simulink model "Automatic_Power_Factor_Improvement_of_Induction_Motor"  (R2022b)
settings: Solver=VariableStepAuto  StartTime=0.0  StopTime=60  RelTol=1e-3
libraries: spsSeriesRLCLoadLib x10, spsIdealSwitchLib x9, spsSeriesRLCBranchLib x4, spsACVoltageSourceLib x1, spsCurrentMeasurementLib x1, spsPowerLib x1, spsVoltageMeasurementLib x1, spspowerguiLib x1
settings Model: PacingRate=0.100000  Creator=saman  LastModifiedBy=MaL!Th
settings SolverCC: ZeroCrossAlgorithm=Adaptive
settings DebuggingCC: IgnoredZcDiagnostic=none  UnconnectedInputMsg=warning  UnconnectedOutputMsg=warning  UnconnectedLineMsg=warning
settings ModelReferenceCC: EnableRefExpFcnMdlSchedulingChecks=on
settings RTWCC: DLArmComputeVersion=19.05

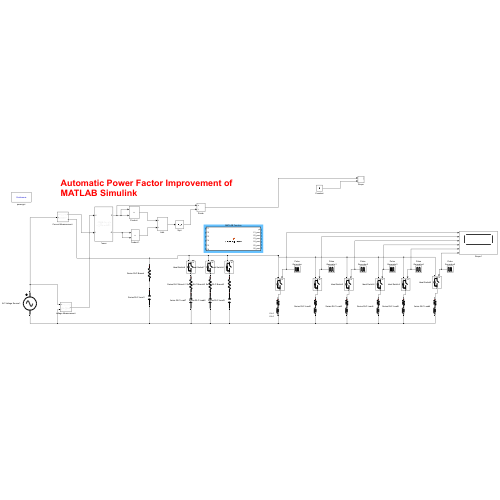
[thumbnail: Simulink's stored preview of the top-level diagram]
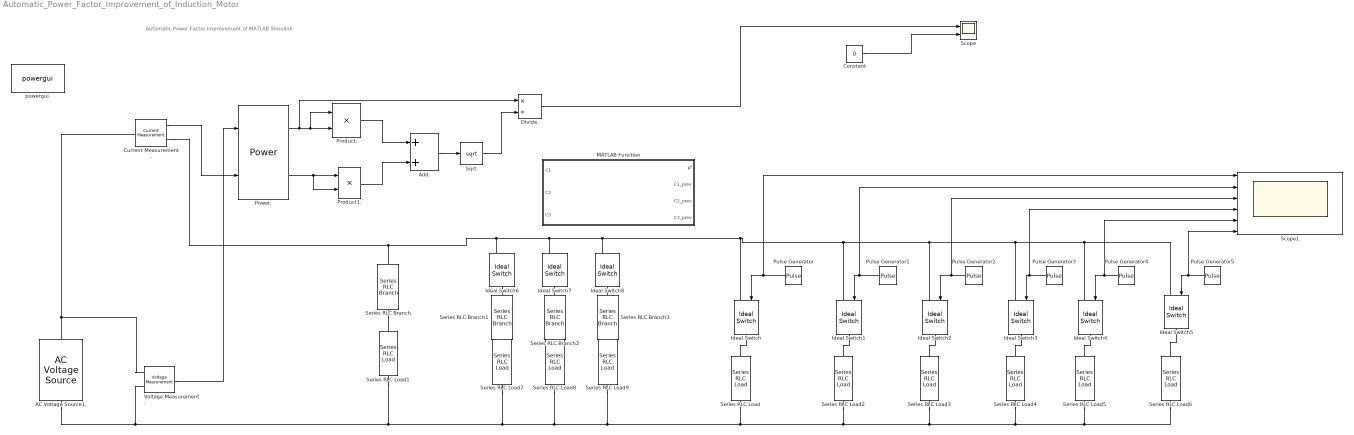
== system Automatic_Power_Factor_Improvement_of_Induction_Motor ==
  note: Automatic Power Factor Improvement of MATLAB Simulink
  AC Voltage Source1. : spsACVoltageSourceLib/AC Voltage Source  Amplitude=311.1  Phase=0  Frequency=50  SampleTime=0  Measurements=None  BusType=swing  Pref=10e3  Qref=0  Qmin=-inf  Qmax=+inf
  Add. : Sum
  Constant : Constant  Value=0
  Current Measurement. : spsCurrentMeasurementLib/Current Measurement  PhasorSimulation=off  OutputType=Complex  PSBequivalent=0
  Divide. : Product  Inputs=*/
  Ideal Switch{,1..8} (9 alike) : spsIdealSwitchLib/Ideal Switch  Ron=0.001  Lon=0  IC=0  Rs=1e5  Cs=inf  Measurements=off
  MATLAB Function : MATLAB Function  TreatAsAtomicUnit=on
  Power. : spsPowerLib/Power  Freq=50  Vinit=[1, 0]  Iinit=[1, 0]  Ts=0
  Product. : Product
  Product1. : Product
  Pulse Generator : DiscretePulseGenerator  PulseType=Time based  Period=70  PulseWidth=14.28  PhaseDelay=50
  Pulse Generator1 : DiscretePulseGenerator  PulseType=Time based  Period=70  PulseWidth=14.28  PhaseDelay=40
  Pulse Generator2 : DiscretePulseGenerator  PulseType=Time based  Period=70  PulseWidth=14.28  PhaseDelay=30
  Pulse Generator3 : DiscretePulseGenerator  PulseType=Time based  Period=70  PulseWidth=14.28  PhaseDelay=20
  Pulse Generator4 : DiscretePulseGenerator  PulseType=Time based  Period=70  PulseWidth=14.28  PhaseDelay=10
  Pulse Generator5 : DiscretePulseGenerator  PulseType=Time based  Period=70  PulseWidth=14.28
  Scope : Scope  NumInputPorts=2
  Scope1 : Scope  NumInputPorts=6
  Series RLC Branch{,1..3} (4 alike) : spsSeriesRLCBranchLib/Series RLC Branch  LConnTagsString=__new0  RConnTagsString=__new0  BranchType=R  Resistance=0.1  Inductance=1e-3  SetiL0=off  InitialCurrent=0  Capacitance=1e-6  Setx0=off  InitialVoltage=0  Measurements=None
  Series RLC Load : spsSeriesRLCLoadLib/Series RLC Load  LConnTagsString=a  RConnTagsString=__new0  NominalVoltage=220  NominalFrequency=50  ActivePower=45e3  InductivePower=40e3  CapacitivePower=0  Setx0=off  InitialVoltage=0  SetiL0=off  InitialCurrent=0  Measurements=None  LoadType=constant Z
      settings: AttributesFormatString=|
      | \n
      | %<ActivePower>
      | %<InductivePower>
  Series RLC Load1 : spsSeriesRLCLoadLib/Series RLC Load  LConnTagsString=a  RConnTagsString=__new0  NominalVoltage=220  NominalFrequency=50  ActivePower=0  InductivePower=0  CapacitivePower=27e3  Setx0=off  InitialVoltage=0  SetiL0=off  InitialCurrent=0  Measurements=None  LoadType=constant Z
  Series RLC Load2 : spsSeriesRLCLoadLib/Series RLC Load  LConnTagsString=a  RConnTagsString=__new0  NominalVoltage=220  NominalFrequency=50  ActivePower=75e3  InductivePower=68e3  CapacitivePower=0  Setx0=off  InitialVoltage=0  SetiL0=off  InitialCurrent=0  Measurements=None  LoadType=constant Z
      settings: AttributesFormatString=\n
  Series RLC Load3 : spsSeriesRLCLoadLib/Series RLC Load  LConnTagsString=a  RConnTagsString=__new0  NominalVoltage=220  NominalFrequency=50  ActivePower=110e3  InductivePower=88e3  CapacitivePower=0  Setx0=off  InitialVoltage=0  SetiL0=off  InitialCurrent=0  Measurements=None  LoadType=constant Z
      settings: AttributesFormatString=\n
  Series RLC Load4 : spsSeriesRLCLoadLib/Series RLC Load  LConnTagsString=a  RConnTagsString=__new0  NominalVoltage=220  NominalFrequency=50  ActivePower=120e3  InductivePower=90e3  CapacitivePower=0  Setx0=off  InitialVoltage=0  SetiL0=off  InitialCurrent=0  Measurements=None  LoadType=constant Z
      settings: AttributesFormatString=\n
  Series RLC Load5 : spsSeriesRLCLoadLib/Series RLC Load  LConnTagsString=a  RConnTagsString=__new0  NominalVoltage=220  NominalFrequency=50  ActivePower=85e3  InductivePower=64e3  CapacitivePower=0  Setx0=off  InitialVoltage=0  SetiL0=off  InitialCurrent=0  Measurements=None  LoadType=constant Z
      settings: AttributesFormatString=\n
  Series RLC Load6 : spsSeriesRLCLoadLib/Series RLC Load  LConnTagsString=a  RConnTagsString=__new0  NominalVoltage=220  NominalFrequency=50  ActivePower=65e3  InductivePower=58e3  CapacitivePower=0  Setx0=off  InitialVoltage=0  SetiL0=off  InitialCurrent=0  Measurements=None  LoadType=constant Z
      settings: AttributesFormatString=\n
  Series RLC Load7 : spsSeriesRLCLoadLib/Series RLC Load  LConnTagsString=a  RConnTagsString=__new0  NominalVoltage=220  NominalFrequency=50  ActivePower=0  InductivePower=0  CapacitivePower=11e3  Setx0=off  InitialVoltage=0  SetiL0=off  InitialCurrent=0  Measurements=None  LoadType=constant Z
  Series RLC Load8 : spsSeriesRLCLoadLib/Series RLC Load  LConnTagsString=a  RConnTagsString=__new0  NominalVoltage=220  NominalFrequency=50  ActivePower=0  InductivePower=0  CapacitivePower=7e3  Setx0=off  InitialVoltage=0  SetiL0=off  InitialCurrent=0  Measurements=None  LoadType=constant Z
  Series RLC Load9 : spsSeriesRLCLoadLib/Series RLC Load  LConnTagsString=a  RConnTagsString=__new0  NominalVoltage=220  NominalFrequency=50  ActivePower=0  InductivePower=0  CapacitivePower=9e3  Setx0=off  InitialVoltage=0  SetiL0=off  InitialCurrent=0  Measurements=None  LoadType=constant Z
  Sqrt. : Sqrt
  Voltage Measurement. : spsVoltageMeasurementLib/Voltage Measurement  PhasorSimulation=off  OutputType=Complex  PSBequivalent=0
  powergui. : spspowerguiLib/powergui  Priority=1  SimulationMode=Continuous  SampleTime=50e-6  frequency=60  Iterations=50  frequencyindice=50  Pbase=100e6  ErrMax=1e-4  UnitsV=kV  UnitsW=MW  buscounter=0  FunctionMessages=off  echomessages=off  EnableUseOfTLC=off  CurrentSourceSwitches=off  DisableSnubberDevices=off  DisableRonSwitches=off  DisableVfSwitches=off  DisplayEquations=off  AutomaticDiscreteSolvers=off  SolverType=Tustin/Backward Euler (TBE)  Interpol=off  ExternalGateDelay=off  methode=off  Ts=100  x0status=blocks  SPID=on  SwTol=0  HookPort=off  NonlinearTolerance=1e-4  nMaxIteration=100  ContinueOnMaxIteration=off  RestoreLinks=warning  ResistiveCurrentMeasurement=off  Frange=[0:2:500]  Ylog=off  Xlog=on  ShowGrid=off  save=off  variable=ZData  structure=0  ZoomFFT=off  StartTime=0.0  cycles=1  DisplayStyle=1  fundamental=60  FreqAxis=off  MaxFrequency=1000  frequencyindicesteady=1  RmsSteady=1  display=off
  wires:
  Product./1 -> Add./1
  Current Measurement./1 -> Power./2
  Sqrt./1 -> Divide./2
  Voltage Measurement./1 -> Power./1
  Power./1 -> Divide./1, Product./1, Product./2
  Product1./1 -> Add./2
  Add./1 -> Sqrt./1
  Power./2 -> Product1./2, Product1./1
  Pulse Generator/1 -> Scope1/1, Ideal Switch/1
  Pulse Generator1/1 -> Scope1/2, Ideal Switch1/1
  Pulse Generator2/1 -> Scope1/3, Ideal Switch2/1
  Pulse Generator3/1 -> Scope1/4, Ideal Switch3/1
  Pulse Generator4/1 -> Scope1/5, Ideal Switch4/1
  Pulse Generator5/1 -> Scope1/6, Ideal Switch5/1
  Divide./1 -> Scope/1
  Constant/1 -> Scope/2
  connections:
  Voltage Measurement./LConn1 -- AC Voltage Source1./RConn1 -- Current Measurement./LConn1
  Ideal Switch/LConn1 -- Ideal Switch6/LConn1 -- Series RLC Branch/LConn1 -- Current Measurement./RConn1 -- Ideal Switch7/LConn1 -- Ideal Switch8/LConn1 -- Ideal Switch5/LConn1 -- Ideal Switch4/LConn1 -- Ideal Switch3/LConn1 -- Ideal Switch2/LConn1 -- Ideal Switch1/LConn1
  AC Voltage Source1./LConn1 -- Voltage Measurement./LConn2 -- Series RLC Load1/RConn1 -- Series RLC Load7/RConn1 -- Series RLC Load9/RConn1 -- Series RLC Load6/RConn1 -- Series RLC Load5/RConn1 -- Series RLC Load4/RConn1 -- Series RLC Load3/RConn1 -- Series RLC Load2/RConn1 -- Series RLC Load/RConn1 -- Series RLC Load8/RConn1
  Series RLC Load/LConn1 -- Ideal Switch/RConn1
  Series RLC Load2/LConn1 -- Ideal Switch1/RConn1
  Series RLC Load3/LConn1 -- Ideal Switch2/RConn1
  Series RLC Load4/LConn1 -- Ideal Switch3/RConn1
  Series RLC Load5/LConn1 -- Ideal Switch4/RConn1
  Series RLC Load6/LConn1 -- Ideal Switch5/RConn1
  Series RLC Branch/RConn1 -- Series RLC Load1/LConn1
  Series RLC Load7/LConn1 -- Series RLC Branch1/RConn1
  Series RLC Branch2/RConn1 -- Series RLC Load8/LConn1
  Series RLC Branch3/RConn1 -- Series RLC Load9/LConn1
  Ideal Switch6/RConn1 -- Series RLC Branch1/LConn1
  Ideal Switch7/RConn1 -- Series RLC Branch2/LConn1
  Series RLC Branch3/LConn1 -- Ideal Switch8/RConn1

== matlab function Automatic_Power_Factor_Improvement_of_Induction_Motor/MATLAB Function ==
  data: pf input; C1 output; C1_prev input; C2_prev input; C3_prev input; C2 output; C3 output
function [C1, C2, C3] = switch_capacitors(pf, C1_prev, C2_prev, C3_prev)
%#codegen

% Hysteresis thresholds
on_threshold = 0.93;
off_threshold = 1.00;

% Initialize outputs with previous states
C1 = C1_prev;
C2 = C2_prev;
C3 = C3_prev;


% Hysteresis switching logic
if pf < on_threshold
    % PF is low → switch ON capacitors progressively
    if C1 == 0
        C1 = 1;
    elseif C2 == 0
        C2 = 1;
    elseif C3 == 0
        C3 = 1;
    end
elseif pf > off_threshold
    % PF is high → switch OFF capacitors progressively
    if C3 == 1
        C3 = 0;
    elseif C2 == 1
        C2 = 0;
    elseif C1 == 1
        C1 = 0;
 
    end
end

end
